simulink model "AFDNFSmodelSPA"  (Simulink 9.0)
settings: Solver=ode45  StartTime=0.0  StopTime=100  FixedStep=1e-3  RelTol=1e-6  EnableMultiTasking=on
InitFcn:
  | run('Methods/AFDSimInit')
values from neighbouring files (symbols this model uses):
  nfs = TransferFunction('Plot','true')    [Main.m]    (also in NFSDatabase.sldd = SI
                Imperial
                28184.4409185639)
undefined symbols (not defined in the file or in its folder): desired, F, K_lat, K_long, Kobsvlat, Kobsvlong, lat, latsys, Light, long, longsys, MIL, Newton, Raphson, sigbuilder_block
libraries: aerolibwind2 x2, sharedutil x1
(part 1 of 3)
settings Model: Creator=AHKh PC  LastModifiedBy=AHKh
settings SolverCC: ZeroCrossAlgorithm=Adaptive  AutoInsertRateTranBlk=on
settings DataIOCC: SignalLoggingSaveFormat=ModelDataLogs  SaveOutput=off
settings OptimizationCC: ExpressionDepthLimit=2147483647
settings DebuggingCC: SolverPrmCheckMsg=warning  FcnCallInpInsideContextMsg=warning  StateNameClashWarn=warning
settings GRTTargetCC: GeneratePreprocessorConditionals=Disable all

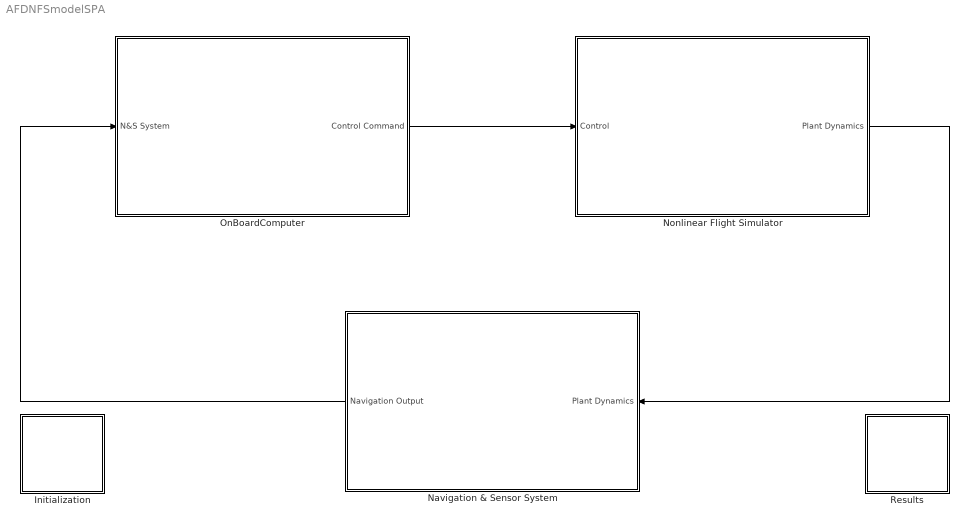
== system AFDNFSmodelSPA ==
  Initialization : Subsystem
      settings: OpenFcn=|
      | % edit('Methods/AFDSimInit.m')
      | !NFSData/NFS Data.xlsx
      mask Display: image(imread('iData/Initialization'))
  Navigation & Sensor System : Subsystem
      mask Display: image(imread('iData/NavigationSystem'))
  Nonlinear Flight Simulator : Subsystem
      mask Display: image(imread('iData/LockheedMartinVARIOUS'));
  OnBoardComputer : Subsystem
      mask Display: image(imread('iData/OnBoardComputerESAPathfinder'));
  Results : Subsystem
      settings: OpenFcn=|
      | cd 'Methods';
      | Plotter(ned_position,euler_angles,control_commands,tout)
      | cd ..
      mask Display: image(imread('iData/Initialization'))
  wires:
  OnBoardComputer/1(Control Command) -> Nonlinear Flight Simulator/1(Control)
  Navigation & Sensor System/1(Navigation Output) -> OnBoardComputer/1(N&S System)
  Nonlinear Flight Simulator/1(Plant Dynamics) -> Navigation & Sensor System/1(Plant Dynamics)

== system AFDNFSmodelSPA/Initialization ==

== system AFDNFSmodelSPA/Navigation & Sensor System ==
  Plant Dynamics : Inport
  Navigation Output : Outport
  wires:
  Plant Dynamics/1 -> Navigation Output/1

== system AFDNFSmodelSPA/Nonlinear Flight Simulator ==
  Control : Inport
  6DoF Nonlinear Flight Equations of Motion (Rigid Body) : Subsystem
  Aerodynamics : Subsystem
  Ground1 : Ground
  Initialization : Subsystem
  Mux : Mux  Inputs=7
  Plot : Subsystem
  Scope : Scope
  Scope1 : Scope
  Scope4 : Scope
  Plant Dynamics : Outport
  wires:
  Aerodynamics/1(Forces (Body)) -> 6DoF Nonlinear Flight Equations of Motion (Rigid Body)/1(Forces (F) (Body)), Scope1/1
  Aerodynamics/2(Moments (Body)) -> Scope4/1, 6DoF Nonlinear Flight Equations of Motion (Rigid Body)/2(Moments (M) (Body))
  6DoF Nonlinear Flight Equations of Motion (Rigid Body)/1(Linear Velocity (Body)) -> Aerodynamics/1(Linear Velocity), Mux/1, Plot/1(Linear Velocity (Body))
  Initialization/3(Initial Inertia tensor) -> 6DoF Nonlinear Flight Equations of Motion (Rigid Body)/5(Inertia Tensor (I))
  Initialization/4(Inertia tensor Change Rate) -> 6DoF Nonlinear Flight Equations of Motion (Rigid Body)/6(Inertia Tensor Change Rate (Idot))
  Control/1 -> Aerodynamics/3(Control)
  Initialization/2(Mass Consumption Rate) -> 6DoF Nonlinear Flight Equations of Motion (Rigid Body)/4(Mass Consumption Rate)
  Initialization/1(Initial Mass) -> 6DoF Nonlinear Flight Equations of Motion (Rigid Body)/3(Initial Mass)
  Initialization/5(Initial Linear Velocity Vector) -> 6DoF Nonlinear Flight Equations of Motion (Rigid Body)/7(Initial Linear  Velocity Vector)
  Initialization/6(Initial Angular Velocity Vector) -> 6DoF Nonlinear Flight Equations of Motion (Rigid Body)/8(Initial Angular  Velocity Vector)
  Initialization/7(Initial Euler Angles) -> 6DoF Nonlinear Flight Equations of Motion (Rigid Body)/9(Initial Euler Angles)
  6DoF Nonlinear Flight Equations of Motion (Rigid Body)/2(Angular Velocity (Body)) -> Aerodynamics/2(Angular Velocity), Mux/2, Plot/2(Angular Velocity (Body))
  6DoF Nonlinear Flight Equations of Motion (Rigid Body)/4(Angular Acceleration (Body)) -> Mux/4, Plot/4(Angular Acceleration (Body))
  Initialization/8(Initial Location (NED)) -> 6DoF Nonlinear Flight Equations of Motion (Rigid Body)/10(Initial Location (NED))
  6DoF Nonlinear Flight Equations of Motion (Rigid Body)/3(Linear Acceleration (Body)) -> Mux/3, Plot/3(Linear Acceleration (Body))
  6DoF Nonlinear Flight Equations of Motion (Rigid Body)/7(Velocity (NED)) -> Mux/7, Plot/7(Velocity (NED))
  Ground1/1 -> Scope/1
  6DoF Nonlinear Flight Equations of Motion (Rigid Body)/6(Position (NED)) -> Aerodynamics/5(Position), Mux/6, Plot/6(Position (NED))
  6DoF Nonlinear Flight Equations of Motion (Rigid Body)/5(Euler Angles) -> Aerodynamics/4(Attitute), Mux/5, Plot/5(Euler Angles)
  Mux/1 -> Plant Dynamics/1
  6DoF Nonlinear Flight Equations of Motion (Rigid Body)/8(T_BI) -> Aerodynamics/6(T_BI)

== system AFDNFSmodelSPA/OnBoardComputer ==
  N&S System : Inport
  Control System : Subsystem
  Guidance Algorithm : Subsystem
  Control Command : Outport
  wires:
  N&S System/1 -> Control System/2(N&S System), Guidance Algorithm/1(N&S System)
  Guidance Algorithm/1(Guidance Command) -> Control System/1(Guidance)
  Control System/1(Control Command) -> Control Command/1

== system AFDNFSmodelSPA/Results ==

== system AFDNFSmodelSPA/Nonlinear Flight Simulator/6DoF Nonlinear Flight Equations of Motion (Rigid Body) ==
  Forces (F) (Body) : Inport
  Moments (M) (Body) : Inport  Port=2  PortDimensions=[3,1]
  Initial Mass : Inport  Port=3
  Mass Consumption Rate : Inport  Port=4
  Inertia Tensor (I) : Inport  Port=5
  Inertia Tensor Change Rate (Idot) : Inport  Port=6
  Initial Linear  Velocity Vector : Inport  Port=7
  Initial Angular  Velocity Vector : Inport  Port=8
  Initial Euler Angles : Inport  Port=9
  Initial Location (NED) : Inport  Port=10
  Angular Velocity Integrator (Body) : Integrator  InitialConditionSource=external  InitialCondition=nfs.angularvel0
  AngularAcceleration(Omegadot) : Subsystem
  Euler angles & Direction Cosine : Subsystem
  Linear Acceleration(Vdot) : Subsystem
  Linear Velocity Integrator (Body) : Integrator  InitialConditionSource=external  InitialCondition=nfs.crusevelvec  ContinuousStateAttributes='BodyVelocity'
  Mass Int : Integrator  InitialConditionSource=external  InitialCondition=nfs.crusevelvec  ContinuousStateAttributes='BodyVelocity'
  Saturation1 : Saturate  UpperLimit=500  LowerLimit=-500
  Saturation2 : Saturate  UpperLimit=500  LowerLimit=-500
  Terminator : Terminator  Commented=on
  Linear Velocity (Body) : Outport
  Angular Velocity (Body) : Outport  Port=2
  Linear Acceleration (Body) : Outport  Port=3
  Angular Acceleration (Body) : Outport  Port=4
  Euler Angles : Outport  Port=5
  Position (NED) : Outport  Port=6
  Velocity (NED) : Outport  Port=7
  T_BI : Outport  Port=8
  wires:
  Initial Mass/1 -> Mass Int/2
  Mass Int/1 -> Linear Acceleration(Vdot)/2(Mass (m))
  Mass Consumption Rate/1 -> Linear Acceleration(Vdot)/3(Mass Reduction Rate (mdot)), Mass Int/1
  Linear Velocity Integrator (Body)/1 -> Saturation1/1  "uvw"
  Angular Velocity Integrator (Body)/1 -> Saturation2/1  "pqr"
  Inertia Tensor (I)/1 -> AngularAcceleration(Omegadot)/3(Inertia Tensor (I))
  Inertia Tensor Change Rate (Idot)/1 -> AngularAcceleration(Omegadot)/4(Inertia Tensor Change Rate (Idot))
  Euler angles & Direction Cosine/1(Direction Cosine Matrix (T_BI)) -> T_BI/1
  Initial Location (NED)/1 -> Euler angles & Direction Cosine/3(Initial Location (NED))
  Forces (F) (Body)/1 -> Linear Acceleration(Vdot)/1(Forces (F))
  Linear Acceleration(Vdot)/1(Linear Acceleration (Vdot)) -> Linear Acceleration (Body)/1, Linear Velocity Integrator (Body)/1
  Initial Linear  Velocity Vector/1 -> Linear Velocity Integrator (Body)/2
  Initial Angular  Velocity Vector/1 -> Angular Velocity Integrator (Body)/2
  AngularAcceleration(Omegadot)/1(Angular Acceleration (Omegadot)) -> Angular Velocity Integrator (Body)/1, Angular Acceleration (Body)/1
  [LinearVelocity] -> Linear Acceleration(Vdot)/4(Linear Velocities (V))
  [AngularVelocity] -> Linear Acceleration(Vdot)/5(Angular Rates (omega))
  Moments (M) (Body)/1 -> AngularAcceleration(Omegadot)/1(Moments (M))
  [AngularVelocity] -> AngularAcceleration(Omegadot)/2(Angular Rates (omega))
  Initial Euler Angles/1 -> Euler angles & Direction Cosine/2(Initial Euler Angles)
  Euler angles & Direction Cosine/4(Velocity (NED)) -> Velocity (NED)/1
  Euler angles & Direction Cosine/2(Euler Angles) -> Euler Angles/1
  Euler angles & Direction Cosine/3(Position (NED)) -> Position (NED)/1
  Saturation1/1 -> Linear Velocity (Body)/1, [LinearVelocity], Euler angles & Direction Cosine/1(Linear Velocity)
  Saturation2/1 -> Angular Velocity (Body)/1, [AngularVelocity], Euler angles & Direction Cosine/4(Angular Velocities)

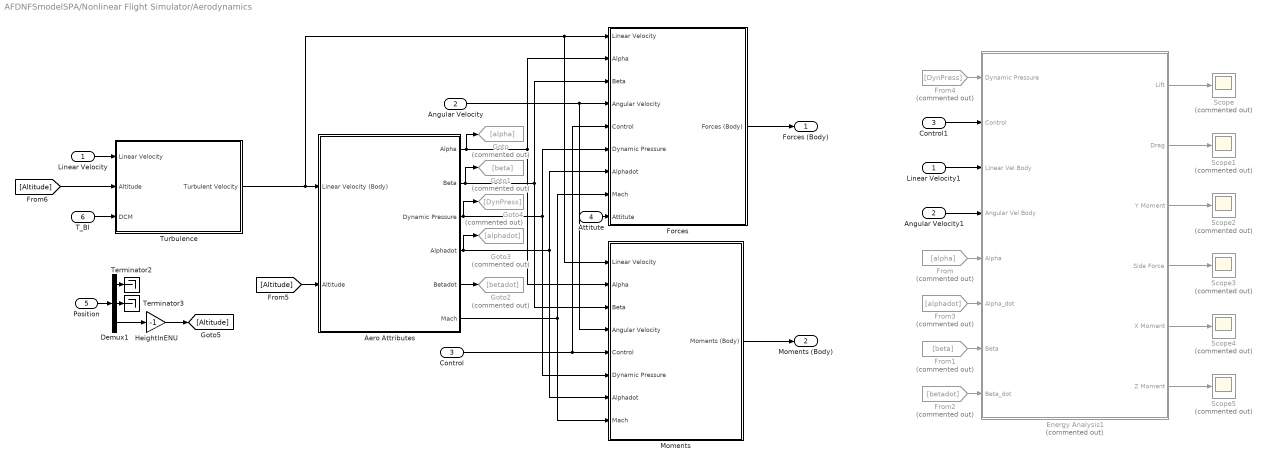
== system AFDNFSmodelSPA/Nonlinear Flight Simulator/Aerodynamics ==
  Linear Velocity : Inport
  Angular Velocity : Inport  Port=2
  Control : Inport  Port=3
  Attitute : Inport  Port=4  PortDimensions=[3,1]
  Position : Inport  Port=5
  T_BI : Inport  Port=6
  Aero Attributes : Subsystem
  Angular Velocity1 : InportShadow  Port=2
  Control1 : InportShadow  Port=3
  Demux1 : Demux  Outputs=3
  Energy Analysis1 : Subsystem  Commented=on  mask{ae=nfs}
      mask prompts: ae "Aero Coefficients"
  Forces : Subsystem
  From : From  Commented=on  GotoTag=alpha
  From1 : From  Commented=on  GotoTag=beta
  From2 : From  Commented=on  GotoTag=betadot
  From3 : From  Commented=on  GotoTag=alphadot
  From4 : From  Commented=on  GotoTag=DynPress
  Goto : Goto  Commented=on  GotoTag=alpha
  Goto1 : Goto  Commented=on  GotoTag=beta
  Goto2 : Goto  Commented=on  GotoTag=betadot
  Goto3 : Goto  Commented=on  GotoTag=alphadot
  Goto4 : Goto  Commented=on  GotoTag=DynPress
  HeightInENU : Gain  Gain=-1  SaturateOnIntegerOverflow=on  OutDataTypeStr=Inherit: Same as input  ParamDataTypeStr=Inherit: Same as input
  Linear Velocity1 : InportShadow
  Moments : Subsystem
  Scope{,1..5} (6 alike) : Scope  Commented=on
  Terminator2 : Terminator
  Terminator3 : Terminator
  Turbulence : Subsystem
  Forces (Body) : Outport
  Moments (Body) : Outport  Port=2
  wires:
  Attitute/1 -> Forces/9(Attitute)
  Forces/1(Forces (Body)) -> Forces (Body)/1
  Demux1/2 -> Terminator3/1
  Demux1/1 -> Terminator2/1
  Demux1/3 -> HeightInENU/1
  Position/1 -> Demux1/1
  Moments/1(Moments (Body)) -> Moments (Body)/1
  Control/1 -> Forces/5(Control), Moments/5(Control)
  Angular Velocity/1 -> Forces/4(Angular Velocity), Moments/4(Angular Velocity)
  Turbulence/1(Turbulent Velocity) -> Forces/1(Linear Velocity), Moments/1(Linear Velocity), Aero Attributes/1(Linear Velocity (Body))
  Aero Attributes/5(Betadot) -> Goto2/1
  Aero Attributes/6(Mach) -> Moments/8(Mach), Forces/8(Mach)
  Aero Attributes/3(Dynamic Pressure) -> Goto4/1, Moments/6(Dynamic Pressure), Forces/6(Dynamic Pressure)
  Aero Attributes/4(Alphadot) -> Goto3/1, Moments/7(Alphadot), Forces/7(Alphadot)
  Aero Attributes/2(Beta) -> Goto1/1, Moments/3(Beta), Forces/3(Beta)
  Aero Attributes/1(Alpha) -> Goto/1, Forces/2(Alpha), Moments/2(Alpha)
  From2/1 -> Energy Analysis1/8(Beta_dot)
  From/1 -> Energy Analysis1/5(Alpha)
  From3/1 -> Energy Analysis1/6(Alpha_dot)
  From1/1 -> Energy Analysis1/7(Beta)
  Control1/1 -> Energy Analysis1/2(Control)
  From4/1 -> Energy Analysis1/1(Dynamic Pressure)
  Linear Velocity1/1 -> Energy Analysis1/3(Linear Vel Body)
  Angular Velocity1/1 -> Energy Analysis1/4(Angular Vel Body)
  Energy Analysis1/1(Lift) -> Scope/1
  Energy Analysis1/2(Drag) -> Scope1/1
  Energy Analysis1/3(Y Moment) -> Scope2/1
  Energy Analysis1/4(Side Force) -> Scope3/1
  Energy Analysis1/5(X Moment) -> Scope4/1
  Energy Analysis1/6(Z Moment) -> Scope5/1
  HeightInENU/1 -> [Altitude]
  [Altitude] -> Aero Attributes/2(Altitude)
  Linear Velocity/1 -> Turbulence/1(Linear Velocity)
  [Altitude] -> Turbulence/2(Altitude)
  T_BI/1 -> Turbulence/3(DCM)

== system AFDNFSmodelSPA/Nonlinear Flight Simulator/Initialization ==
  Constant : Constant  Value=nfs.mass
  Constant1 : Constant  Value=nfs.consumprate
  Constant2 : Constant  Value=nfs.I
  Constant3 : Constant  Value=zeros(3)
  Constant4 : Constant  Value=nfs.crusevelvec
  Constant6 : Constant  Value=nfs.angularvel0
  Constant7 : Constant  Value=nfs.attitude0
  Constant8 : Constant  Value=nfs.initialpos
  Reshape1 : Reshape
  Reshape2 : Reshape  OutputDimensionality=Customize  OutputDimensions=[3,3]
  Reshape3 : Reshape  OutputDimensionality=Customize  OutputDimensions=[3,3]
  Reshape{4,6..8} (4 alike) : Reshape  OutputDimensionality=Column vector (2-D)
  Reshape5 : Reshape
  Initial Mass : Outport
  Mass Consumption Rate : Outport  Port=2
  Initial Inertia tensor : Outport  Port=3
  Inertia tensor Change Rate : Outport  Port=4
  Initial Linear Velocity Vector : Outport  Port=5
  Initial Angular Velocity Vector : Outport  Port=6
  Initial Euler Angles : Outport  Port=7
  Initial Location (NED) : Outport  Port=8
  wires:
  Constant/1 -> Reshape5/1
  Constant1/1 -> Reshape1/1
  Constant2/1 -> Reshape2/1
  Constant3/1 -> Reshape3/1
  Constant4/1 -> Reshape4/1
  Constant6/1 -> Reshape6/1
  Constant7/1 -> Reshape7/1
  Constant8/1 -> Reshape8/1
  Reshape5/1 -> Initial Mass/1
  Reshape1/1 -> Mass Consumption Rate/1
  Reshape2/1 -> Initial Inertia tensor/1
  Reshape3/1 -> Inertia tensor Change Rate/1
  Reshape4/1 -> Initial Linear Velocity Vector/1
  Reshape6/1 -> Initial Angular Velocity Vector/1
  Reshape7/1 -> Initial Euler Angles/1
  Reshape8/1 -> Initial Location (NED)/1

== system AFDNFSmodelSPA/Nonlinear Flight Simulator/Plot ==
  Linear Velocity (Body) : Inport
  Angular Velocity (Body) : Inport  Port=2
  Linear Acceleration (Body) : Inport  Port=3
  Angular Acceleration (Body) : Inport  Port=4
  Euler Angles : Inport  Port=5  PortDimensions=3
  Position (NED) : Inport  Port=6  PortDimensions=3
  Velocity (NED) : Inport  Port=7
  Angular Acceleration - (Body) : Scope
  Angular Velocity - (Body) : Scope
  Euler Angles1 : Scope
  Euler Angles2 : InportShadow  Port=5  PortDimensions=3
  Gain{,1..2,5} (4 alike) : Gain  Gain=180/pi
  Gain3 : Gain  Gain=[1,1,-1]'
  Gain4 : Gain  Gain=[1,1,-1]'
  Linear Acceleration - (Body) : Scope
  Linear Velocity - (Body) : Scope
  Position (NED)1 : InportShadow  Port=6  PortDimensions=3
  Position - (NED) : Scope
  To Workspace : ToWorkspace  VariableName=ned_position  SampleTime=-1
  To Workspace1 : ToWorkspace  VariableName=euler_angles  SampleTime=-1
  Velocity - (NED) : Scope
  wires:
  Gain/1 -> Euler Angles1/1
  Euler Angles/1 -> Gain/1
  Position (NED)/1 -> Gain3/1
  Linear Velocity (Body)/1 -> Linear Velocity - (Body)/1
  Angular Velocity (Body)/1 -> Gain2/1
  Linear Acceleration (Body)/1 -> Linear Acceleration - (Body)/1
  Angular Acceleration (Body)/1 -> Gain1/1
  Velocity (NED)/1 -> Velocity - (NED)/1
  Gain1/1 -> Angular Acceleration - (Body)/1
  Gain2/1 -> Angular Velocity - (Body)/1
  Gain3/1 -> Position - (NED)/1
  Position (NED)1/1 -> Gain4/1
  Gain4/1 -> To Workspace/1
  Euler Angles2/1 -> Gain5/1
  Gain5/1 -> To Workspace1/1

== system AFDNFSmodelSPA/OnBoardComputer/Control System ==
  Guidance : Inport
  N&S System : Inport  Port=2
  Constant2 : Constant  Value=[0 0 0 0]'
  Demux : Demux
  Ground2 : Ground  Commented=on
  LQR : Subsystem
  Manual Switch1 : ManualSwitch
  Mux : Mux
  Scope : Scope
  Sum : Sum  Inputs=++|
  Terminator{,1..3} (4 alike) : Terminator  Commented=on
  Terminator4 : Terminator
  To Workspace1 : ToWorkspace  VariableName=control_commands  SampleTime=-1
  Trim Offset +  Reference Excitation : Subsystem
  Unfinished Controllers (State-Feedback) : Subsystem  Commented=on
  Control Command : Outport
  wires:
  Sum/1 -> Scope/1, Control Command/1, To Workspace1/1
  [delta_e] -> Mux/1
  [delta_f] -> Mux/2
  [delta_a] -> Mux/3
  [delta_r] -> Mux/4
  Trim Offset +  Reference Excitation/1(Trim) -> Sum/1
  Mux/1 -> Manual Switch1/1
  Constant2/1 -> Manual Switch1/2
  Manual Switch1/1 -> Sum/2
  Ground2/1 -> Unfinished Controllers (State-Feedback)/1(Reference Input)
  Unfinished Controllers (State-Feedback)/1(dE) -> Terminator/1
  Unfinished Controllers (State-Feedback)/2(dF) -> Terminator1/1
  Unfinished Controllers (State-Feedback)/3(dA) -> Terminator2/1
  Unfinished Controllers (State-Feedback)/4(dR) -> Terminator3/1
  Guidance/1 -> Terminator4/1
  N&S System/1 -> LQR/1(N&S System)
  Demux/1 -> [delta_e]
  Demux/2 -> [delta_f]
  Demux/3 -> [delta_a]
  Demux/4 -> [delta_r]
  LQR/1(Control Command) -> Demux/1

== system AFDNFSmodelSPA/OnBoardComputer/Guidance Algorithm ==
  note: There is no guidance algorithm yet!
  N&S System : Inport
  Constant : Constant  Value=desired.pitch
  Constant1 : Constant  Value=[nfs.crusevelvec(1); nfs.crusevelvec(3)]
  Constant2 : Constant  Value=nfs.crusevelvec(2)
  Demux : Demux  Outputs=7
  Mux : Mux  Inputs=2
  Mux1 : Mux  Inputs=3
  Mux2 : Mux  Inputs=3
  Selector : Selector  InputPortWidth=3  IndexOptions=Index vector (dialog)  Indices=[2]  OutputSizes=1
  Selector1 : Selector  InputPortWidth=3  IndexOptions=Index vector (dialog)  Indices=[2]  OutputSizes=1
  Selector2 : Selector  InputPortWidth=3  IndexOptions=Index vector (dialog)  Indices=[2]  OutputSizes=1
  Selector3 : Selector  InputPortWidth=3  IndexOptions=Index vector (dialog)  Indices=[1 3]  OutputSizes=1
  Selector4 : Selector  InputPortWidth=3  IndexOptions=Index vector (dialog)  Indices=[1 3]  OutputSizes=1
  Selector5 : Selector  InputPortWidth=3  IndexOptions=Index vector (dialog)  Indices=[1 3]  OutputSizes=1
  Sum : Sum  Inputs=|+-
  Sum1 : Sum  Inputs=-+|
  Sum2 : Sum  Inputs=|+-
  Terminator{1..4} (4 alike) : Terminator
  Guidance Command : Outport
  wires:
  N&S System/1 -> Demux/1
  Demux/1 -> Selector3/1, Selector1/1  "Linear Velocity (Body)"
  Demux/3 -> Terminator1/1  "Linear Acceleration (Body)"
  Demux/4 -> Terminator2/1  "Angular Acceleration (Body)"
  Demux/7 -> Terminator4/1  "Velocity (NED)"
  Demux/2 -> Selector/1, Selector4/1  "Angular Velocity (Body)"
  Demux/6 -> Terminator3/1  "Position (NED)"
  Demux/5 -> Selector2/1, Selector5/1  "Euler Angles"
  Mux/1 -> Guidance Command/1
  Mux1/1 -> Mux/1
  Mux2/1 -> Mux/2
  Selector/1 -> Mux1/2  "q"
  Selector4/1 -> Mux2/2  "p & r"
  Selector5/1 -> Mux2/3  "phi & psi"
  Selector2/1 -> Sum/1  "Theta"
  Sum/1 -> Mux1/3
  Constant/1 -> Sum/2
  Sum1/1 -> Mux1/1
  Selector3/1 -> Sum1/2  "u & w"
  Constant1/1 -> Sum1/1
  Selector1/1 -> Sum2/1  "v"
  Sum2/1 -> Mux2/1
  Constant2/1 -> Sum2/2

== system AFDNFSmodelSPA/Nonlinear Flight Simulator/6DoF Nonlinear Flight Equations of Motion (Rigid Body)/AngularAcceleration(Omegadot) ==
  Moments (M) : Inport  PortDimensions=[3,1]
  Angular Rates (omega) : Inport  Port=2  PortDimensions=[3,1]
  Inertia Tensor (I) : Inport  Port=3
  Inertia Tensor Change Rate (Idot) : Inport  Port=4
  Angular Rates (omega)1 : InportShadow  Port=2  PortDimensions=[3,1]
  Cross Product : Subsystem  mask(Cross Product){}
      mask help: Calculate the cross product of two 3-by-1 vectors.
      mask Display:
      | text(.5,.5,'Cross\nProduct\nC = AxB', ...
      | 	'HorizontalAlignment','Center',...
      | 	'VerticalAlignment','middle')
  Inertia Tensor (I)1 : InportShadow  Port=3
  Product1 : Product  Inputs=**  Multiplication=Matrix(*)  SaturateOnIntegerOverflow=on  OutDataTypeStr=Inherit: Same as first input
  Product3 : Product  Inputs=**  Multiplication=Matrix(*)  SaturateOnIntegerOverflow=on  OutDataTypeStr=Inherit: Same as first input
  Product4 : Product  Inputs=/*  Multiplication=Matrix(*)  SaturateOnIntegerOverflow=on  OutDataTypeStr=Inherit: Same as first input
  Sum1 : Sum  Inputs=|+-  SaturateOnIntegerOverflow=on
  Sum3 : Sum  Inputs=|+-  SaturateOnIntegerOverflow=on
  Angular Acceleration (Omegadot) : Outport
  wires:
  Product3/1 -> Sum1/2
  Product1/1 -> Cross Product/2(B)
  Cross Product/1(C) -> Sum3/2
  Sum1/1 -> Sum3/1
  Sum3/1 -> Product4/2
  Product4/1 -> Angular Acceleration (Omegadot)/1
  Inertia Tensor (I)1/1 -> Product4/1
  Moments (M)/1 -> Sum1/1
  Inertia Tensor Change Rate (Idot)/1 -> Product3/1
  Angular Rates (omega)/1 -> Cross Product/1(A), Product3/2
  Angular Rates (omega)1/1 -> Product1/2
  Inertia Tensor (I)/1 -> Product1/1

== system AFDNFSmodelSPA/Nonlinear Flight Simulator/6DoF Nonlinear Flight Equations of Motion (Rigid Body)/Euler angles & Direction Cosine ==
  Linear Velocity : Inport  PortDimensions=[3,1]
  Initial Euler Angles : Inport  Port=2
  Initial Location (NED) : Inport  Port=3  PortDimensions=[3,1]
  Angular Velocities : Inport  Port=4
  Constant : Constant
  Euler Angles Int : Integrator  InitialConditionSource=external  InitialCondition=nfs.attitude0
  Euler angles Calculation : Subsystem
  If : If  IfExpression=u1(3)>= 0  ShowElse=off
  If Action Subsystem : Subsystem  TreatAsAtomicUnit=on
  Position Integrator : Integrator  InitialConditionSource=external  InitialCondition=[0,0,nfs.attitude0]
  Rotation Angles to DCM : Subsystem
  Selector : Selector  InputPortWidth=3  IndexOptions=Index vector (dialog)  Indices=[3 2 1]  OutputSizes=1
  Transform from Body to Inertial axes : Subsystem
      mask Display: disp('T_IB')
  Transpose : Math  Operator=transpose  SaturateOnIntegerOverflow=on
  Direction Cosine Matrix (T_BI) : Outport  PortDimensions=[3,3]
  Euler Angles : Outport  Port=2
  Position (NED) : Outport  Port=3  PortDimensions=[3,1]
  Velocity (NED) : Outport  Port=4  PortDimensions=[3,1]
  wires:
  Initial Euler Angles/1 -> Euler Angles Int/2
  Rotation Angles to DCM/1(DCM) -> Transpose/1, Direction Cosine Matrix (T_BI)/1
  Angular Velocities/1 -> Euler angles Calculation/1(Angular Velocities)
  Selector/1 -> Rotation Angles to DCM/1("[R1,R2,R3]")
  Transpose/1 -> Transform from Body to Inertial axes/1(Transformation Matrix)
  Linear Velocity/1 -> Transform from Body to Inertial axes/2(Position Vector)
  Initial Location (NED)/1 -> Position Integrator/2
  Euler Angles Int/1 -> Euler Angles/1, Selector/1, Euler angles Calculation/2(Euler Angles)
  Transform from Body to Inertial axes/1(Ve) -> Velocity (NED)/1, Position Integrator/1
  Position Integrator/1 -> Position (NED)/1, If/1
  Euler angles Calculation/1(Euler Rates) -> Euler Angles Int/1
  If/1 -> If Action Subsystem/Action
  Constant/1 -> If Action Subsystem/1(Simulation Termination)

== system AFDNFSmodelSPA/Nonlinear Flight Simulator/6DoF Nonlinear Flight Equations of Motion (Rigid Body)/Linear Acceleration(Vdot) ==
  Forces (F) : Inport  PortDimensions=[3,1]
  Mass (m) : Inport  Port=2
  Mass Reduction Rate (mdot) : Inport  Port=3
  Linear Velocities (V) : Inport  Port=4  PortDimensions=[3,1]
  Angular Rates (omega) : Inport  Port=5
  Cross Product : Subsystem  mask(Cross Product){}
      mask help: Calculate the cross product of two 3-by-1 vectors.
      mask Display:
      | text(.5,.5,'Cross\nProduct\nC = AxB', ...
      | 	'HorizontalAlignment','Center',...
      | 	'VerticalAlignment','middle')
  Linear Velocities (V)1 : InportShadow  Port=4  PortDimensions=[3,1]
  Mass (m)1 : InportShadow  Port=2
  Product : Product  Inputs=*/  SaturateOnIntegerOverflow=on  OutDataTypeStr=Inherit: Same as first input
  Product1 : Product  Inputs=*/  SaturateOnIntegerOverflow=on  OutDataTypeStr=Inherit: Same as first input
  Product3 : Product  Inputs=**  SaturateOnIntegerOverflow=on  OutDataTypeStr=Inherit: Same as first input
  Sum1 : Sum  Inputs=|+-  SaturateOnIntegerOverflow=on
  Sum3 : Sum  Inputs=|+-  SaturateOnIntegerOverflow=on
  Linear Acceleration (Vdot) : Outport
  wires:
  Mass (m)/1 -> Product/2
  Product/1 -> Sum1/1
  Mass Reduction Rate (mdot)/1 -> Product1/1
  Mass (m)1/1 -> Product1/2
  Product1/1 -> Product3/1
  Product3/1 -> Sum1/2
  Sum1/1 -> Sum3/1
  Cross Product/1(C) -> Sum3/2
  Linear Velocities (V)/1 -> Product3/2
  Forces (F)/1 -> Product/1
  Sum3/1 -> Linear Acceleration (Vdot)/1
  Angular Rates (omega)/1 -> Cross Product/1(A)
  Linear Velocities (V)1/1 -> Cross Product/2(B)

== system AFDNFSmodelSPA/Nonlinear Flight Simulator/Aerodynamics/Aero Attributes ==
  Linear Velocity (Body) : Inport  PortDimensions=[3,1]
  Altitude : Inport  Port=2
  Beta Saturation : Saturate  UpperLimit=5*pi/11  LowerLimit=-5*pi/11
  Beta Saturation1 : Saturate  UpperLimit=1  LowerLimit=-1
  Demux1 : Demux  Outputs=3
  Derivative1 : Derivative
  Derivative2 : Derivative
  Dynamic Pressure Calc : Subsystem
  Linear Velocity (Body)1 : InportShadow  PortDimensions=[3,1]
  Reshape13 : Reshape
  Scope{1..3,7} (4 alike) : Scope
  Subsystem : Subsystem
  Trigonometric Function2 : Trigonometry  Operator=atan
  Trigonometric Function3 : Trigonometry  Operator=asin
  Velocity Magnitude : Subsystem
  w/u1 : Product  Inputs=/*  SaturateOnIntegerOverflow=on  InputSameDT=on  OutDataTypeStr=Inherit: Same as first input
  w/u2 : Product  Inputs=*/  SaturateOnIntegerOverflow=on  InputSameDT=on  OutDataTypeStr=Inherit: Same as first input
  w/u3 : Product  Inputs=*/  SaturateOnIntegerOverflow=on  InputSameDT=on  OutDataTypeStr=Inherit: Same as first input
  Alpha : Outport
  Beta : Outport  Port=2
  Dynamic Pressure : Outport  Port=3
  Alphadot : Outport  Port=4
  Betadot : Outport  Port=5
  Mach : Outport  Port=6
  wires:
  Beta Saturation1/1 -> Alphadot/1, Scope1/1
  Subsystem/2(Air Density) -> Dynamic Pressure Calc/1(Air Density)
  Subsystem/1(Speed of Sound) -> w/u3/2
  Velocity Magnitude/1(Velocity Magnitude) -> w/u3/1, w/u2/2
  Reshape13/1 -> Mach/1
  Derivative2/1 -> Betadot/1, Scope3/1  "Betadot"
  Beta Saturation/1 -> Beta/1, Scope2/1
  Derivative1/1 -> Beta Saturation1/1
  Dynamic Pressure Calc/1(Dynamic Pressure) -> Dynamic Pressure/1
  Linear Velocity (Body)1/1 -> Dynamic Pressure Calc/2(Linear Velocity (Body))
  Altitude/1 -> Subsystem/1(Height)
  w/u3/1 -> Reshape13/1
  Trigonometric Function3/1 -> Beta Saturation/1, Derivative2/1
  Trigonometric Function2/1 -> Derivative1/1, Alpha/1, Scope7/1
  w/u2/1 -> Trigonometric Function3/1
  w/u1/1 -> Trigonometric Function2/1
  Demux1/3 -> w/u1/2  "W"
  Demux1/2 -> w/u2/1  "V"
  Demux1/1 -> w/u1/1  "U"
  Linear Velocity (Body)/1 -> Velocity Magnitude/1(Velocity), Demux1/1

== system AFDNFSmodelSPA/Nonlinear Flight Simulator/Aerodynamics/Energy Analysis1 ==
  Dynamic Pressure : Inport
  Control : Inport  Port=2
  Linear Vel Body : Inport  Port=3
  Angular Vel Body : Inport  Port=4
  Alpha : Inport  Port=5
  Alpha_dot : Inport  Port=6
  Beta : Inport  Port=7
  Beta_dot : Inport  Port=8
  Angular Vel Body0 : InportShadow  Port=4
  Constant{1..2,5,8} (4 alike) : Constant  Value=0
  Constant3 : Constant  Value=ae.refarea
  Constant4 : Constant  Value=ae.span
  Constant6 : Constant  Value=ae.refarea
  Constant9 : Constant  Value=ae.meanchord
  Control3 : InportShadow  Port=2
  Demux1 : Demux
  Demux2 : Demux
  Dynamic Pressure2 : InportShadow
  Lateral-Directional1 : Subsystem
  Linear Vel Body2 : InportShadow  Port=3
  Longitudinal1 : Subsystem
  Lift : Outport
  Drag : Outport  Port=2
  Y Moment : Outport  Port=3
  Side Force : Outport  Port=4
  X Moment : Outport  Port=5
  Z Moment : Outport  Port=6
  wires:
  Lateral-Directional1/1(fy) -> Side Force/1
  Lateral-Directional1/2(l) -> X Moment/1
  Lateral-Directional1/3(n) -> Z Moment/1
  Longitudinal1/2(m) -> Y Moment/1
  Longitudinal1/1(D) -> Drag/1
  Longitudinal1/3(L) -> Lift/1
  Dynamic Pressure/1 -> Lateral-Directional1/1(Dynamic Pressure)
  Constant3/1 -> Lateral-Directional1/2(S)
  Linear Vel Body/1 -> Lateral-Directional1/4(Linear Vel Body)
  Angular Vel Body0/1 -> Lateral-Directional1/5(Angular Vel Body)
  Constant5/1 -> Lateral-Directional1/13(iH)
  Constant4/1 -> Lateral-Directional1/3(b)
  Beta/1 -> Lateral-Directional1/6(Beta)
  Beta_dot/1 -> Lateral-Directional1/7(Beta_dot)
  Demux1/1 -> Lateral-Directional1/8(DeltaElevator)
  Demux1/2 -> Lateral-Directional1/9(DeltaFlap)
  Demux1/4 -> Lateral-Directional1/11(DeltaRudder)
  Demux1/3 -> Lateral-Directional1/10(DeltaAileron)
  Constant1/1 -> Lateral-Directional1/12(DeltaThrust)
  Control/1 -> Demux1/1
  Constant6/1 -> Longitudinal1/2(S)
  Alpha/1 -> Longitudinal1/6(Alpha)
  Angular Vel Body/1 -> Longitudinal1/4(Angular Vel)
  Dynamic Pressure2/1 -> Longitudinal1/1(Dynamic Pressure)
  Linear Vel Body2/1 -> Longitudinal1/3(Linear Vel Body)
  Constant9/1 -> Longitudinal1/5(c_bar)
  Alpha_dot/1 -> Longitudinal1/7(Alpha_dot)
  Constant8/1 -> Longitudinal1/13(iH)
  Constant2/1 -> Longitudinal1/12(Delta_Thrust)
  Demux2/4 -> Longitudinal1/11(DeltaRudder)
  Demux2/2 -> Longitudinal1/9(DeltaFlap)
  Demux2/3 -> Longitudinal1/10(DeltaAileron)
  Demux2/1 -> Longitudinal1/8(DeltaElevator)
  Control3/1 -> Demux2/1

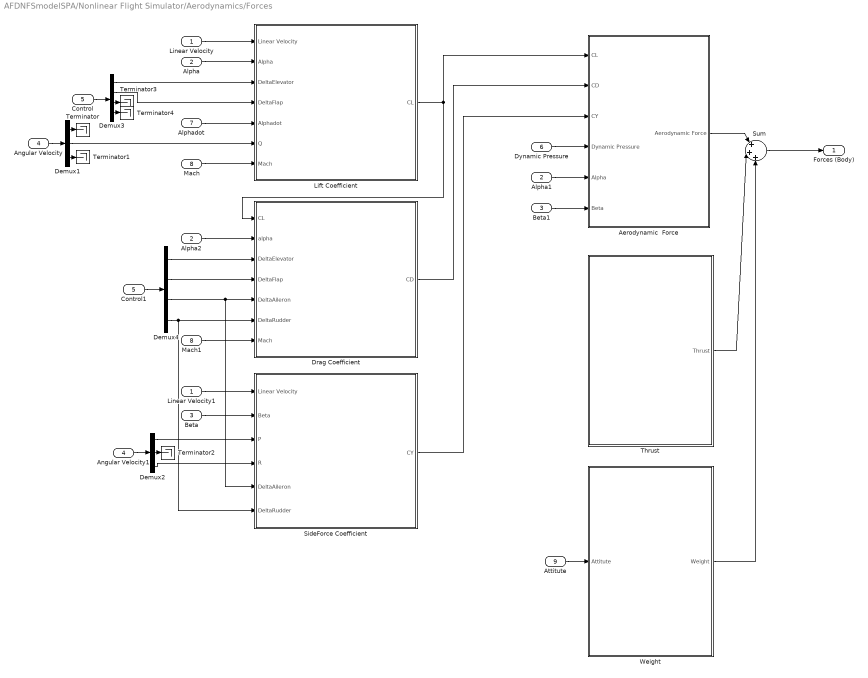
== system AFDNFSmodelSPA/Nonlinear Flight Simulator/Aerodynamics/Forces ==
  Linear Velocity : Inport  PortDimensions=[3,1]
  Alpha : Inport  Port=2  PortDimensions=1
  Beta : Inport  Port=3
  Angular Velocity : Inport  Port=4  PortDimensions=[3,1]
  Control : Inport  Port=5  PortDimensions=[4,1]
  Dynamic Pressure : Inport  Port=6
  Alphadot : Inport  Port=7  PortDimensions=1
  Mach : Inport  Port=8
  Attitute : Inport  Port=9  PortDimensions=[3,1]
  Aerodynamic  Force : Subsystem
  Alpha1 : InportShadow  Port=2  PortDimensions=1
  Alpha2 : InportShadow  Port=2  PortDimensions=1
  Angular Velocity1 : InportShadow  Port=4  PortDimensions=[3,1]
  Beta1 : InportShadow  Port=3
  Control1 : InportShadow  Port=5  PortDimensions=[4,1]
  Demux1 : Demux  Outputs=3
  Demux2 : Demux  Outputs=3
  Demux3 : Demux
  Demux4 : Demux
  Drag Coefficient : Subsystem  mask{cD0=nfs.aero.cD0}
  Lift Coefficient : Subsystem  mask{cL0=nfs.aero.cL0, meanchord=nfs.meanchord}
      mask prompts: meanchord "Mean Aerodynamic Chord"
  Linear Velocity1 : InportShadow  PortDimensions=[3,1]
  Mach1 : InportShadow  Port=8
  SideForce Coefficient : Subsystem
  Sum : Sum  Inputs=|+|+|+
  Terminator{,1..4} (5 alike) : Terminator
  Thrust : Subsystem
  Weight : Subsystem
  Forces (Body) : Outport
  wires:
  Thrust/1(Thrust) -> Sum/2
  Weight/1(Weight) -> Sum/3
  Attitute/1 -> Weight/1(Attitute)
  Sum/1 -> Forces (Body)/1
  Aerodynamic  Force/1(Aerodynamic Force) -> Sum/1
  Alpha/1 -> Lift Coefficient/2(Alpha)
  Mach1/1 -> Drag Coefficient/7(Mach)
  Mach/1 -> Lift Coefficient/7(Mach)
  Alphadot/1 -> Lift Coefficient/5(Alphadot)
  Beta1/1 -> Aerodynamic  Force/6(Beta)
  Alpha1/1 -> Aerodynamic  Force/5(Alpha)
  Dynamic Pressure/1 -> Aerodynamic  Force/4(Dynamic Pressure)
  Demux4/4 -> SideForce Coefficient/6(DeltaRudder), Drag Coefficient/6(DeltaRudder)
  Demux4/3 -> SideForce Coefficient/5(DeltaAileron), Drag Coefficient/5(DeltaAileron)
  Demux4/2 -> Drag Coefficient/4(DeltaFlap)
  Demux4/1 -> Drag Coefficient/3(DeltaElevator)
  Control1/1 -> Demux4/1
  Demux3/4 -> Terminator4/1
  Demux3/3 -> Terminator3/1
  Demux3/2 -> Lift Coefficient/4(DeltaFlap)
  Demux3/1 -> Lift Coefficient/3(DeltaElevator)
  Control/1 -> Demux3/1
  Demux2/2 -> Terminator2/1
  Demux2/3 -> SideForce Coefficient/4(R)
  Demux2/1 -> SideForce Coefficient/3(P)
  Angular Velocity1/1 -> Demux2/1
  Demux1/3 -> Terminator1/1
  Demux1/1 -> Terminator/1
  Angular Velocity/1 -> Demux1/1
  Demux1/2 -> Lift Coefficient/6(Q)
  Beta/1 -> SideForce Coefficient/2(Beta)
  Linear Velocity1/1 -> SideForce Coefficient/1(Linear Velocity)
  Linear Velocity/1 -> Lift Coefficient/1(Linear Velocity)
  SideForce Coefficient/1(CY) -> Aerodynamic  Force/3(CY)
  Drag Coefficient/1(CD) -> Aerodynamic  Force/2(CD)
  Lift Coefficient/1(CL) -> Aerodynamic  Force/1(CL), Drag Coefficient/1(CL)
  Alpha2/1 -> Drag Coefficient/2(alpha)

== system AFDNFSmodelSPA/Nonlinear Flight Simulator/Aerodynamics/Moments ==
  Linear Velocity : Inport  PortDimensions=[3,1]
  Alpha : Inport  Port=2
  Beta : Inport  Port=3
  Angular Velocity : Inport  Port=4  PortDimensions=[3,1]
  Control : Inport  Port=5
  Dynamic Pressure : Inport  Port=6
  Alphadot : Inport  Port=7
  Mach : Inport  Port=8
  "Aerodynamic Moment " : Subsystem
  Alpha1 : InportShadow  Port=2
  Beta1 : InportShadow  Port=3
  Beta2 : InportShadow  Port=3
  Demux1 : Demux  Outputs=3
  Demux2 : Demux
  Linear Velocity1 : InportShadow  PortDimensions=[3,1]
  Linear Velocity2 : InportShadow  PortDimensions=[3,1]
  Pitch Moment Coefficient : Subsystem
  Roll Moment Coefficient : Subsystem
  Yaw Moment Coefficient : Subsystem
  Moments (Body) : Outport
  wires:
  Demux2/2 -> Pitch Moment Coefficient/5(DeltaFlap)
  Demux2/1 -> Pitch Moment Coefficient/4(DeltaElevator)
  Demux2/4 -> Yaw Moment Coefficient/6(DeltaRudder), Roll Moment Coefficient/6(DeltaRudder)
  Demux2/3 -> Yaw Moment Coefficient/5(DeltaAileron), Roll Moment Coefficient/5(DeltaAileron)
  Control/1 -> Demux2/1
  Mach/1 -> Pitch Moment Coefficient/7(Mach)
  Alphadot/1 -> Pitch Moment Coefficient/6(Alphadot)
  Demux1/2 -> Pitch Moment Coefficient/3(Q)
  Demux1/3 -> Yaw Moment Coefficient/4(R), Roll Moment Coefficient/4(R)
  Demux1/1 -> Yaw Moment Coefficient/3(P), Roll Moment Coefficient/3(P)
  Angular Velocity/1 -> Demux1/1
  Beta1/1 -> Yaw Moment Coefficient/2(beta)
  Beta/1 -> Roll Moment Coefficient/2(Beta)
  Alpha/1 -> Pitch Moment Coefficient/2(Alpha)
  Dynamic Pressure/1 -> "Aerodynamic Moment "/4(Dynamic Pressure)
  Linear Velocity2/1 -> Yaw Moment Coefficient/1(Linear Velocity)
  Linear Velocity1/1 -> Pitch Moment Coefficient/1(Linear Velocity)
  Linear Velocity/1 -> Roll Moment Coefficient/1(Linear Velocity)
  "Aerodynamic Moment "/1(Aerodynamic Moment) -> Moments (Body)/1
  Yaw Moment Coefficient/1(Cn) -> "Aerodynamic Moment "/3(Cn)
  Pitch Moment Coefficient/1(Cm) -> "Aerodynamic Moment "/2(Cm)
  Roll Moment Coefficient/1(Cl) -> "Aerodynamic Moment "/1(Cl)
  Alpha1/1 -> "Aerodynamic Moment "/5(Alpha)
  Beta2/1 -> "Aerodynamic Moment "/6(Beta)

== system AFDNFSmodelSPA/Nonlinear Flight Simulator/Aerodynamics/Turbulence ==
  Linear Velocity : Inport
  Altitude : Inport  Port=2
  DCM : Inport  Port=3
  Altitude1 : InportShadow  Port=2
  DCM1 : InportShadow  Port=3
  Dryden Wind Turbulence Model  (Continuous (+q +r)) : aerolibwind2/Dryden Wind Turbulence Model  (Continuous (+q -r))  units=Metric (MKS)  spec=MIL-F-8785C  model=Continuous Dryden (+q +r)  W20=15  Wdeg=0  TurbProb=10^-2 - Light  L_high=533.4  Wingspan=nfs.span  ts=0.001  Seed=[23341 23342 23343 23344]  T_on=on
      settings: SourceProductName=Aerospace Blockset
  Linear Velocity1 : InportShadow
  Linear Velocity2 : InportShadow
  Linear Velocity3 : InportShadow
  Manual Switch : ManualSwitch
  Manual Switch1 : ManualSwitch  CurrentSetting=0
  Sum : Sum  Inputs=++|
  Terminator : Terminator
  Terminator1 : Terminator
  Terminator2 : Terminator
  Velocity Magnitude : Subsystem
  Velocity Magnitude1 : Subsystem
  Von Karman Wind Turbulence Model  (Continuous (+q +r)) : aerolibwind2/Dryden Wind Turbulence Model  (Continuous (+q -r))  units=Metric (MKS)  spec=MIL-F-8785C  model=Continuous Von Karman (+q +r)  W20=15  Wdeg=0  TurbProb=10^-2 - Light  L_high=762  Wingspan=10.3  ts=0.001  Seed=[23341 23342 23343 23344]  T_on=on
      settings: SourceProductName=Aerospace Blockset
  Turbulent Velocity : Outport
  wires:
  Linear Velocity/1 -> Velocity Magnitude/1(Velocity)
  Altitude/1 -> Dryden Wind Turbulence Model  (Continuous (+q +r))/1
  DCM/1 -> Dryden Wind Turbulence Model  (Continuous (+q +r))/3
  Velocity Magnitude/1(Velocity Magnitude) -> Dryden Wind Turbulence Model  (Continuous (+q +r))/2
  Dryden Wind Turbulence Model  (Continuous (+q +r))/2 -> Terminator/1
  Sum/1 -> Manual Switch1/1
  Linear Velocity1/1 -> Velocity Magnitude1/1(Velocity)
  Altitude1/1 -> Von Karman Wind Turbulence Model  (Continuous (+q +r))/1
  Velocity Magnitude1/1(Velocity Magnitude) -> Von Karman Wind Turbulence Model  (Continuous (+q +r))/2
  DCM1/1 -> Von Karman Wind Turbulence Model  (Continuous (+q +r))/3
  Von Karman Wind Turbulence Model  (Continuous (+q +r))/2 -> Terminator1/1
  Dryden Wind Turbulence Model  (Continuous (+q +r))/1 -> [DrydenVel]
  Von Karman Wind Turbulence Model  (Continuous (+q +r))/1 -> [KarmanVel]
  [KarmanVel] -> Manual Switch/2
  [DrydenVel] -> Manual Switch/1
  Manual Switch/1 -> Sum/2
  Linear Velocity2/1 -> Sum/1
  Manual Switch1/1 -> Turbulent Velocity/1
  Linear Velocity3/1 -> Manual Switch1/2

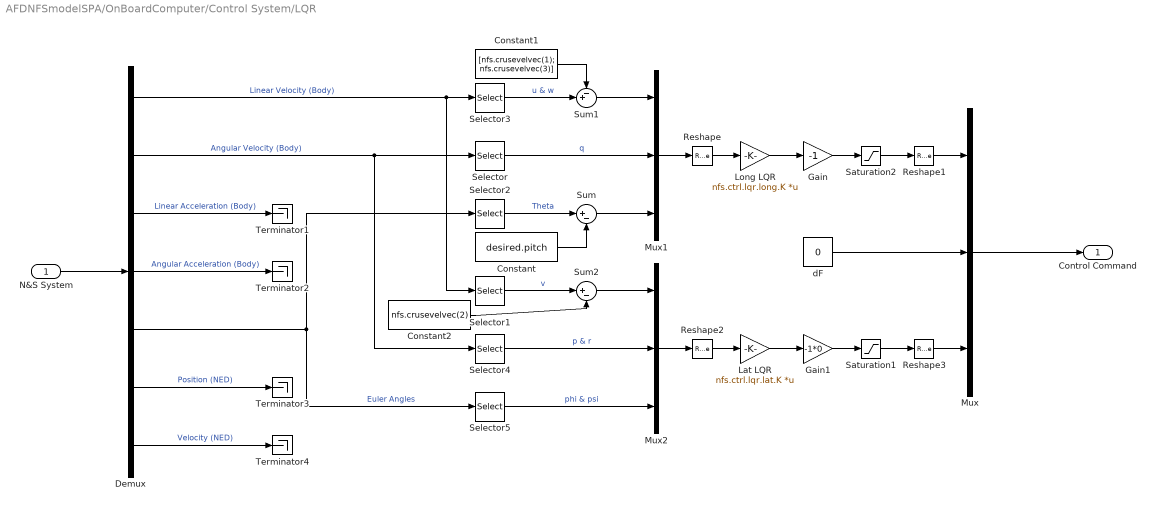
== system AFDNFSmodelSPA/OnBoardComputer/Control System/LQR ==
  N&S System : Inport
  Constant : Constant  Value=desired.pitch
  Constant1 : Constant  Value=[nfs.crusevelvec(1); nfs.crusevelvec(3)]
  Constant2 : Constant  Value=nfs.crusevelvec(2)
  Demux : Demux  Outputs=7
  Gain : Gain  Gain=-1
  Gain1 : Gain  Gain=-1*0
  Lat LQR : Gain  Gain=nfs.ctrl.lqr.lat.K  Multiplication=Matrix(K*u)
  Long LQR : Gain  Gain=nfs.ctrl.lqr.long.K  Multiplication=Matrix(K*u)
  Mux : Mux  Inputs=3
  Mux1 : Mux  Inputs=3
  Mux2 : Mux  Inputs=3
  Reshape : Reshape  OutputDimensionality=Customize  OutputDimensions=[4,1]
  Reshape1 : Reshape  OutputDimensionality=Customize
  Reshape2 : Reshape  OutputDimensionality=Customize  OutputDimensions=[5,1]
  Reshape3 : Reshape  OutputDimensionality=Customize  OutputDimensions=[2,1]
  Saturation1 : Saturate  UpperLimit=deg2rad(15)  LowerLimit=-deg2rad(15)
  Saturation2 : Saturate  UpperLimit=deg2rad(15)  LowerLimit=-deg2rad(15)
  Selector : Selector  InputPortWidth=3  IndexOptions=Index vector (dialog)  Indices=[2]  OutputSizes=1
  Selector1 : Selector  InputPortWidth=3  IndexOptions=Index vector (dialog)  Indices=[2]  OutputSizes=1
  Selector2 : Selector  InputPortWidth=3  IndexOptions=Index vector (dialog)  Indices=[2]  OutputSizes=1
  Selector3 : Selector  InputPortWidth=3  IndexOptions=Index vector (dialog)  Indices=[1 3]  OutputSizes=1
  Selector4 : Selector  InputPortWidth=3  IndexOptions=Index vector (dialog)  Indices=[1 3]  OutputSizes=1
  Selector5 : Selector  InputPortWidth=3  IndexOptions=Index vector (dialog)  Indices=[1 3]  OutputSizes=1
  Sum : Sum  Inputs=|+-
  Sum1 : Sum  Inputs=-+|
  Sum2 : Sum  Inputs=|+-
  Terminator{1..4} (4 alike) : Terminator
  dF : Constant  Value=0
  Control Command : Outport
  wires:
  Constant1/1 -> Sum1/1
  Constant2/1 -> Sum2/2
  Sum2/1 -> Mux2/1
  Selector1/1 -> Sum2/1  "v"
  Demux/4 -> Terminator2/1  "Angular Acceleration (Body)"
  Selector5/1 -> Mux2/3  "phi & psi"
  Selector/1 -> Mux1/2  "q"
  Selector4/1 -> Mux2/2  "p & r"
  Demux/1 -> Selector3/1, Selector1/1  "Linear Velocity (Body)"
  Constant/1 -> Sum/2
  Demux/2 -> Selector/1, Selector4/1  "Angular Velocity (Body)"
  Demux/6 -> Terminator3/1  "Position (NED)"
  Sum1/1 -> Mux1/1
  Demux/7 -> Terminator4/1  "Velocity (NED)"
  Demux/5 -> Selector2/1, Selector5/1  "Euler Angles"
  Sum/1 -> Mux1/3
  Demux/3 -> Terminator1/1  "Linear Acceleration (Body)"
  Selector3/1 -> Sum1/2  "u & w"
  Selector2/1 -> Sum/1  "Theta"
  N&S System/1 -> Demux/1
  Mux1/1 -> Reshape/1
  Long LQR/1 -> Gain/1
  Lat LQR/1 -> Gain1/1
  Mux2/1 -> Reshape2/1
  Gain/1 -> Saturation2/1
  dF/1 -> Mux/2
  Gain1/1 -> Saturation1/1
  Mux/1 -> Control Command/1
  Reshape/1 -> Long LQR/1
  Reshape1/1 -> Mux/1
  Reshape2/1 -> Lat LQR/1
  Reshape3/1 -> Mux/3
  Saturation1/1 -> Reshape3/1
  Saturation2/1 -> Reshape1/1

== system AFDNFSmodelSPA/OnBoardComputer/Control System/Trim Offset +  Reference Excitation ==
  Constant1 : Constant  Value=[nfs.trim.delta_e;0;0;0]
  Doublet Generated Signal : Subsystem
  Manual Switch : ManualSwitch
  Manual Switch1 : ManualSwitch  CurrentSetting=0
  Triangular signal span 10 sec : Subsystem
  Trim : Outport
  wires:
  Constant1/1 -> Manual Switch/2
  Doublet Generated Signal/1(Doublet Out) -> Manual Switch1/1
  Triangular signal span 10 sec/1(Tri) -> Manual Switch1/2
  Manual Switch1/1 -> Manual Switch/1
  Manual Switch/1 -> Trim/1

== system AFDNFSmodelSPA/OnBoardComputer/Control System/Unfinished Controllers (State-Feedback) ==
  Reference Input : Inport
  Demux : Demux  Outputs=2
  Demux1 : Demux  Outputs=2
  Full-State Feedback Servo : Subsystem
  Full-State Observer Servo : Subsystem
  Ground : Ground
  Ground1 : Ground
  Ground2 : Ground
  Manual Switch{2,4..6} (4 alike) : ManualSwitch  CurrentSetting=0
  Manual Switch3 : ManualSwitch
  Reduced Order Observer Servo : Subsystem
  Scope : Scope
  Scope1 : Scope
  Terminator : Terminator
  Terminator1 : Terminator
  dE : Outport
  dF : Outport  Port=2
  dA : Outport  Port=3
  dR : Outport  Port=4
  wires:
  Reduced Order Observer Servo/1(Longitudinal Control) -> Terminator/1
  Reduced Order Observer Servo/2(Lateral-Directional Control) -> Terminator1/1
  Full-State Observer Servo/2(Lateral-Directional Control) -> Manual Switch5/2
  Full-State Feedback Servo/1(Longitudinal Control) -> Scope/1, Manual Switch4/1
  Ground1/1 -> Manual Switch3/2
  Ground/1 -> Manual Switch2/2
  Demux/1 -> dE/1
  [U] -> Full-State Observer Servo/2(U)
  Manual Switch5/1 -> Demux1/1
  Manual Switch4/1 -> Demux/1
  Full-State Feedback Servo/2(Lateral-Directional Control) -> Manual Switch5/1
  Demux1/2 -> dR/1
  Reference Input/1 -> Scope1/1, Manual Switch3/1, Manual Switch6/1, Manual Switch2/1
  Manual Switch2/1 -> Full-State Observer Servo/1(States)
  Demux1/1 -> dA/1
  Manual Switch3/1 -> Full-State Feedback Servo/1(States)
  Demux/2 -> dF/1
  Manual Switch6/1 -> Reduced Order Observer Servo/1(States)
  Ground2/1 -> Manual Switch6/2
  Full-State Observer Servo/1(Longitudinal Control) -> Manual Switch4/2

== system AFDNFSmodelSPA/Nonlinear Flight Simulator/6DoF Nonlinear Flight Equations of Motion (Rigid Body)/AngularAcceleration(Omegadot)/Cross Product ==
  A : Inport
  B : Inport  Port=2
  "A " : InportShadow
  "B " : InportShadow  Port=2
  Subsystem2 : Subsystem
  Subsystem3 : Subsystem
  Sum : Sum  Inputs=+|-  SaturateOnIntegerOverflow=on  InputSameDT=on  OutDataTypeStr=Inherit: Same as first input
  C : Outport
  wires:
  Subsystem3/1(Out2) -> Sum/2
  Subsystem2/1(Out1) -> Sum/1
  A/1 -> Subsystem2/1(A)
  B/1 -> Subsystem2/2(B)
  Sum/1 -> C/1
  "A "/1 -> Subsystem3/1(A)
  "B "/1 -> Subsystem3/2(B)

== system AFDNFSmodelSPA/Nonlinear Flight Simulator/6DoF Nonlinear Flight Equations of Motion (Rigid Body)/Euler angles & Direction Cosine/Euler angles Calculation ==
  Angular Velocities : Inport  PortDimensions=[3,1]
  Euler Angles : Inport  Port=2
  Mux1 : Mux  Inputs=[3 3 3]
  Mux2 : Mux  Inputs=3
  phidot : Fcn  Expr=u[1]+(u[2]*u[4]+u[3]*u[7])*(u[5]/u[8])
  psidot : Fcn  Expr=(u[2]*u[4]+u[3]*u[7])/u[8]
  sincos : Trigonometry  Operator=sincos
  thetadot : Fcn  Expr=u[2]*u[7]-u[3]*u[4]
  Euler Rates : Outport  PortDimensions=[3,1]  InitialOutput=0
  wires:
  sincos/2 -> Mux1/3
  sincos/1 -> Mux1/2
  Mux2/1 -> Euler Rates/1
  phidot/1 -> Mux2/1
  thetadot/1 -> Mux2/2
  psidot/1 -> Mux2/3
  Euler Angles/1 -> sincos/1
  Angular Velocities/1 -> Mux1/1
  Mux1/1 -> psidot/1, phidot/1, thetadot/1

== system AFDNFSmodelSPA/Nonlinear Flight Simulator/6DoF Nonlinear Flight Equations of Motion (Rigid Body)/Euler angles & Direction Cosine/If Action Subsystem ==
  Simulation Termination : Inport
  Action Port : ActionPort  ActionType=then
  Stop Simulation : Stop
  wires:
  Simulation Termination/1 -> Stop Simulation/1

== system AFDNFSmodelSPA/Nonlinear Flight Simulator/6DoF Nonlinear Flight Equations of Motion (Rigid Body)/Euler angles & Direction Cosine/Rotation Angles to DCM ==
  "[R1,R2,R3]" : Inport  PortDimensions=3
  Create 3x3 Matrix : sharedutil/Create 3x3 Matrix
  Fcn11 : Fcn  Expr=u(5)*u(4)
  Fcn12 : Fcn  Expr=u(5)*u(1)
  Fcn13 : Fcn  Expr=-u(2)
  Fcn21 : Fcn  Expr=u(3)*u(2)*u(4) - u(6)*u(1)
  Fcn22 : Fcn  Expr=u(3)*u(2)*u(1) + u(6)*u(4)
  Fcn23 : Fcn  Expr=u(3)*u(5)
  Fcn31 : Fcn  Expr=u(6)*u(2)*u(4) + u(3)*u(1)
  Fcn32 : Fcn  Expr=u(6)*u(2)*u(1) - u(3)*u(4)
  Fcn33 : Fcn  Expr=u(6)*u(5)
  Mux : Mux  Inputs=2
  sincos1 : Trigonometry  Operator=sincos
  DCM : Outport  PortDimensions=[3,3]
  wires:
  "[R1,R2,R3]"/1 -> sincos1/1
  Create 3x3 Matrix/1 -> DCM/1
  sincos1/1 -> Mux/1
  sincos1/2 -> Mux/2
  Mux/1 -> Fcn32/1, Fcn33/1, Fcn31/1, Fcn23/1, Fcn22/1, Fcn11/1, Fcn12/1, Fcn13/1, Fcn21/1
  Fcn11/1 -> Create 3x3 Matrix/1
  Fcn12/1 -> Create 3x3 Matrix/2
  Fcn13/1 -> Create 3x3 Matrix/3
  Fcn21/1 -> Create 3x3 Matrix/4
  Fcn31/1 -> Create 3x3 Matrix/7
  Fcn22/1 -> Create 3x3 Matrix/5
  Fcn23/1 -> Create 3x3 Matrix/6
  Fcn32/1 -> Create 3x3 Matrix/8
  Fcn33/1 -> Create 3x3 Matrix/9

== system AFDNFSmodelSPA/Nonlinear Flight Simulator/6DoF Nonlinear Flight Equations of Motion (Rigid Body)/Euler angles & Direction Cosine/Transform from Body to Inertial axes ==
  Transformation Matrix : Inport
  Position Vector : Inport  Port=2
  Product : Product  Multiplication=Matrix(*)  SaturateOnIntegerOverflow=on  InputSameDT=on  OutDataTypeStr=Inherit: Same as first input
  Reshape1 : Reshape  OutputDimensionality=Column vector (2-D)
  Reshape2 : Reshape
  Ve : Outport
  wires:
  Reshape2/1 -> Ve/1
  Reshape1/1 -> Product/2
  Position Vector/1 -> Reshape1/1
  Transformation Matrix/1 -> Product/1
  Product/1 -> Reshape2/1

== system AFDNFSmodelSPA/Nonlinear Flight Simulator/6DoF Nonlinear Flight Equations of Motion (Rigid Body)/Linear Acceleration(Vdot)/Cross Product ==
  A : Inport
  B : Inport  Port=2
  "A " : InportShadow
  "B " : InportShadow  Port=2
  Subsystem2 : Subsystem
  Subsystem3 : Subsystem
  Sum : Sum  Inputs=+|-  SaturateOnIntegerOverflow=on  InputSameDT=on  OutDataTypeStr=Inherit: Same as first input
  C : Outport
  wires:
  Subsystem3/1(Out2) -> Sum/2
  Subsystem2/1(Out1) -> Sum/1
  A/1 -> Subsystem2/1(A)
  B/1 -> Subsystem2/2(B)
  Sum/1 -> C/1
  "A "/1 -> Subsystem3/1(A)
  "B "/1 -> Subsystem3/2(B)

== system AFDNFSmodelSPA/Nonlinear Flight Simulator/Aerodynamics/Aero Attributes/Dynamic Pressure Calc ==
  Air Density : Inport  PortDimensions=1
  Linear Velocity (Body) : Inport  Port=2  PortDimensions=[3 1]
  0.5*rh : Product  SaturateOnIntegerOverflow=on  InputSameDT=on  OutDataTypeStr=Inherit: Same as first input
  Dot Product : DotProduct  InputSameDT=on  OutDataTypeStr=Inherit: Inherit via internal rule
  Gain : Gain  Gain=0.5  SaturateOnIntegerOverflow=on  OutDataTypeStr=Inherit: Same as input  ParamDataTypeStr=Inherit: Same as input
  V^2 : Abs
  Dynamic Pressure : Outport
  wires:
  Dot Product/1 -> V^2/1
  Linear Velocity (Body)/1 -> Dot Product/2, Dot Product/1
  Air Density/1 -> Gain/1
  V^2/1 -> 0.5*rh/1
  Gain/1 -> 0.5*rh/2
  0.5*rh/1 -> Dynamic Pressure/1

== system AFDNFSmodelSPA/Nonlinear Flight Simulator/Aerodynamics/Aero Attributes/Subsystem ==
  Height : Inport
  "(T/T0)^(g/LR) " : Math  Operator=pow  SaturateOnIntegerOverflow=on
  1/T0 : Gain  Gain=1/288.15  SaturateOnIntegerOverflow=on  OutDataTypeStr=Inherit: Same as input  ParamDataTypeStr=Inherit: Same as input
  Altitude of Troposphere : Constant  Value=11000  OutDataTypeStr=Inherit: Inherit via back propagation
  Lapse Rate : Gain  Gain=0.0065  SaturateOnIntegerOverflow=on  OutDataTypeStr=Inherit: Same as input  ParamDataTypeStr=Inherit: Same as input
  Limit  altitude  to Stratosphere : Saturate  UpperLimit=0  LowerLimit=11000-20000
  Limit  altitude  to troposhere : Saturate  UpperLimit=11000  LowerLimit=0
  Product : Product  Inputs=*/  SaturateOnIntegerOverflow=on  InputSameDT=on  OutDataTypeStr=Inherit: Same as first input
  Product1 : Product  Inputs=/*  SaturateOnIntegerOverflow=on  InputSameDT=on  OutDataTypeStr=Inherit: Same as first input
  Product3 : Product  SaturateOnIntegerOverflow=on  InputSameDT=on  OutDataTypeStr=Inherit: Same as first input
  Sea Level  Temperature : Constant  Value=288.15  OutDataTypeStr=Inherit: Inherit via back propagation
  Stratosphere Model : Math  SaturateOnIntegerOverflow=on
  Sum : Sum  Inputs=+-  SaturateOnIntegerOverflow=on  InputSameDT=on  OutDataTypeStr=Inherit: Same as first input
  Sum1 : Sum  Inputs=+-  SaturateOnIntegerOverflow=on  InputSameDT=on  OutDataTypeStr=Inherit: Same as first input
  a : Sqrt  AlgorithmType=Newton-Raphson  SaturateOnIntegerOverflow=on
  g/(L*R) : Constant  Value=9.80665/(0.0065*287.0531)  OutDataTypeStr=Inherit: Inherit via back propagation
  g/R : Gain  Gain=9.80665/287.0531  SaturateOnIntegerOverflow=on  OutDataTypeStr=Inherit: Same as input  ParamDataTypeStr=Inherit: Same as input
  gamma*R : Gain  Gain=1.4*287.0531  SaturateOnIntegerOverflow=on  OutDataTypeStr=Inherit: Same as input  ParamDataTypeStr=Inherit: Same as input
  rho0 : Gain  Gain=1.225  SaturateOnIntegerOverflow=on  OutDataTypeStr=Inherit: Same as input  ParamDataTypeStr=Inherit: Same as input
  Speed of Sound : Outport  PortDimensions=1
  Air Density : Outport  Port=2  PortDimensions=1
  wires:
  g/(L*R)/1 -> "(T/T0)^(g/LR) "/2
  Height/1 -> Limit  altitude  to troposhere/1, Sum/2
  Limit  altitude  to troposhere/1 -> Lapse Rate/1
  Product/1 -> rho0/1
  "(T/T0)^(g/LR) "/1 -> Product/1
  1/T0/1 -> "(T/T0)^(g/LR) "/1, Product/2
  gamma*R/1 -> a/1
  a/1 -> Speed of Sound/1
  Sum1/1 -> gamma*R/1, 1/T0/1, Product1/1
  Lapse Rate/1 -> Sum1/2
  Sea Level  Temperature/1 -> Sum1/1
  rho0/1 -> Product3/1
  Product3/1 -> Air Density/1
  Stratosphere Model/1 -> Product3/2
  g/R/1 -> Product1/2
  Product1/1 -> Stratosphere Model/1
  Altitude of Troposphere/1 -> Sum/1
  Sum/1 -> Limit  altitude  to Stratosphere/1
  Limit  altitude  to Stratosphere/1 -> g/R/1

== system AFDNFSmodelSPA/Nonlinear Flight Simulator/Aerodynamics/Aero Attributes/Velocity Magnitude ==
  Velocity : Inport
  Dot Product : DotProduct  InputSameDT=on  OutDataTypeStr=Inherit: Inherit via internal rule
  Sqrt : Sqrt  SaturateOnIntegerOverflow=on
  Velocity Magnitude : Outport
  wires:
  Sqrt/1 -> Velocity Magnitude/1  "abs(V)"
  Velocity/1 -> Dot Product/2, Dot Product/1
  Dot Product/1 -> Sqrt/1
